simulink model "ISReferenceApplication"  (R2019b)
settings: Solver=VariableStepAuto  StartTime=0.0  StopTime=10.0  RelTol=1e-3
undefined symbols (not defined in the file or in its folder): C_Brake, C_Final, C_Front, C_Middle, C_out_Brake, C_out_Final, C_out_Front, C_out_Middle, Co, Cso, D_out_Brake, D_out_Final, D_out_Front, D_out_Middle, Downshift_Speeds, F, F_Brake, F_Final, F_Front, F_Middle, Fs, G_Brake, G_Final, G_Front, G_Middle, G_sys_Brake, G_sys_Final, G_sys_Front, G_sys_Middle, Gd, Gd_Brake, Gd_Final, Gsd, h, H_Brake, H_Final, H_Front, H_Middle, H_sys_Brake, H_sys_Final, H_sys_Front, H_sys_Middle, Hd, Hd_Brake, Hd_Final, Hsd, JE, JE_Brake, JE_Final, JE_Front, JE_Middle, JEs, JF_part, JF_part_Brake, JF_part_Final, JF_parts, Ld, Ld_Brake, Ld_Final, Ld_Front ... (+21)
libraries: simulink x5, autolibutils x3, sim3dlib x2, vehdynlibviscommon x1
(part 2 of 4)

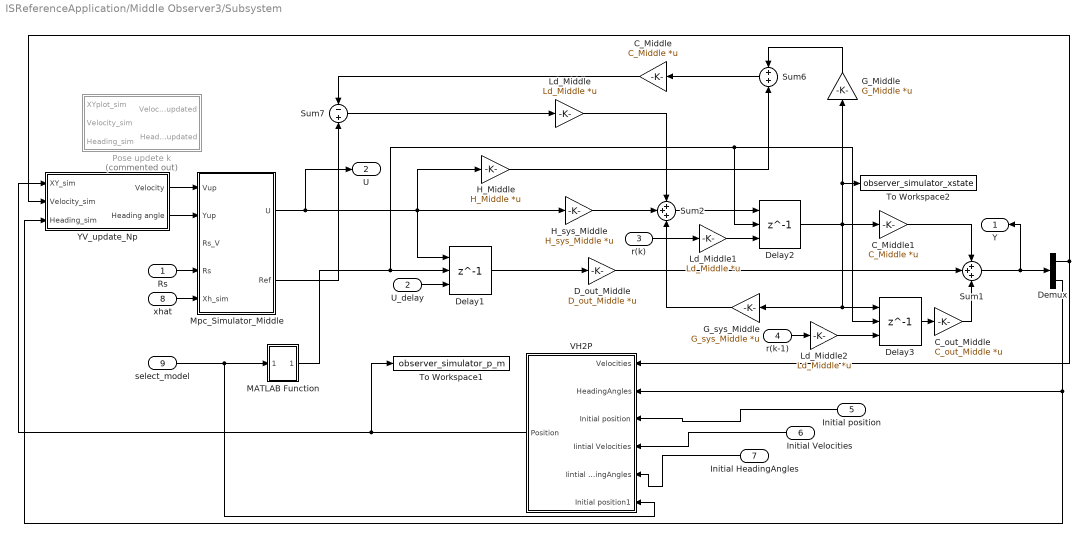
== system ISReferenceApplication/Middle Observer3/Subsystem ==
  Rs : Inport
  U_delay : Inport  Port=2
  r(k) : Inport  Port=3
  r(k-1) : Inport  Port=4
  Initial position : Inport  Port=5
  Initial Velocities : Inport  Port=6
  Initial HeadingAngles : Inport  Port=7
  xhat : Inport  Port=8
  select_model : Inport  Port=9
  C_Middle : Gain  Gain=C_Middle  Multiplication=Matrix(K*u) (u vector)
  C_Middle1 : Gain  Gain=C_Middle  Multiplication=Matrix(K*u) (u vector)
  C_out_Middle : Gain  Gain=C_out_Middle  Multiplication=Matrix(K*u) (u vector)
  D_out_Middle : Gain  Gain=D_out_Middle  Multiplication=Matrix(K*u) (u vector)
  Delay1 : Delay  DelayLength=1  InitialConditionSource=Input port  InitialCondition=0  ExternalReset=Rising  SampleTime=Ts
      settings: InputPortMap=u0,r5,p4
  Delay2 : Delay  DelayLength=1  InitialConditionSource=Input port  InitialCondition=0  ExternalReset=Rising  SampleTime=Ts
      settings: InputPortMap=u0,r5,p4
  Delay3 : Delay  DelayLength=1  InitialConditionSource=Input port  InitialCondition=0  ExternalReset=Rising  SampleTime=Ts
      settings: InputPortMap=u0,r5,p4
  Demux : Demux  Outputs=2
  G_Middle : Gain  Gain=G_Middle  Multiplication=Matrix(K*u) (u vector)
  G_sys_Middle : Gain  Gain=G_sys_Middle  Multiplication=Matrix(K*u) (u vector)
  H_Middle : Gain  Gain=H_Middle  Multiplication=Matrix(K*u) (u vector)
  H_sys_Middle : Gain  Gain=H_sys_Middle  Multiplication=Matrix(K*u) (u vector)
  Ld_Middle : Gain  Gain=Ld_Middle  Multiplication=Matrix(K*u) (u vector)
  Ld_Middle1 : Gain  Gain=Ld_Middle  Multiplication=Matrix(K*u) (u vector)
  Ld_Middle2 : Gain  Gain=Ld_Middle  Multiplication=Matrix(K*u) (u vector)
  MATLAB Function : MATLAB Function  TreatAsAtomicUnit=on
  Mpc_Simulator_Middle : Subsystem
  Pose updete k : Subsystem  Commented=on
  Sum1 : Sum  Inputs=+++
  Sum2 : Sum  Inputs=+++
  Sum6 : Sum
  Sum7 : Sum  Inputs=-+
  To Workspace1 : ToWorkspace  VariableName=observer_simulator_p_m  SampleTime=Ts
  To Workspace2 : ToWorkspace  VariableName=observer_simulator_xstate  SampleTime=Ts
  VH2P : Subsystem
  YV_update_Np : Subsystem  TreatAsAtomicUnit=on
  Y : Outport  VectorParamsAs1DForOutWhenUnconnected=off
  U : Outport  Port=2  VectorParamsAs1DForOutWhenUnconnected=off
  wires:
  MATLAB Function/1(tri) -> Delay1/2, Delay2/2, Delay3/2
  select_model/1 -> MATLAB Function/1(select_model), VH2P/6(Initial position1)
  Initial position/1 -> VH2P/3(Initial position)
  Sum2/1 -> Delay2/1
  Demux/2 -> YV_update_Np/3(Heading_sim), VH2P/2(HeadingAngles)
  Ld_Middle/1 -> Sum2/1
  Sum7/1 -> Ld_Middle/1
  Mpc_Simulator_Middle/2(Ref) -> Sum7/2
  Rs/1 -> Mpc_Simulator_Middle/4(Rs)
  C_out_Middle/1 -> Sum1/3
  G_Middle/1 -> Sum6/1
  C_Middle/1 -> Sum7/1
  Mpc_Simulator_Middle/1(U) -> U/1, H_sys_Middle/1, H_Middle/1, Delay1/1
  H_sys_Middle/1 -> Sum2/2
  G_sys_Middle/1 -> Sum2/3
  Delay3/1 -> C_out_Middle/1
  VH2P/1(Position) -> YV_update_Np/1(XY_sim), To Workspace1/1
  Demux/1 -> YV_update_Np/2(Velocity_sim), VH2P/1(Velocities)
  Delay2/1 -> To Workspace2/1, G_Middle/1, G_sys_Middle/1, Delay3/1, C_Middle1/1
  H_Middle/1 -> Sum6/2
  Sum1/1 -> Y/1, Demux/1
  Sum6/1 -> C_Middle/1
  D_out_Middle/1 -> Sum1/2
  Delay1/1 -> D_out_Middle/1
  C_Middle1/1 -> Sum1/1
  YV_update_Np/2(Heading angle) -> Mpc_Simulator_Middle/2(Yup)
  xhat/1 -> Mpc_Simulator_Middle/5(Xh_sim)
  YV_update_Np/1(Velocity) -> Mpc_Simulator_Middle/1(Vup)
  r(k)/1 -> Ld_Middle1/1
  Ld_Middle1/1 -> Delay2/3
  U_delay/1 -> Delay1/3
  r(k-1)/1 -> Ld_Middle2/1
  Ld_Middle2/1 -> Delay3/3
  Initial Velocities/1 -> VH2P/4(Iintial Velocities)
  Initial HeadingAngles/1 -> VH2P/5(Iintial HeadingAngles)

== system ISReferenceApplication/Passenger Vehicle/Body, Suspension, Wheels ==
  note: 1) Add Subsystem or Model blocks as valid variant choices.
      | 2) You cannot connect blocks at this level. At simulation, connectivity is automatically
      | determined, based on the active variant and port name matching.
  WindXYZ : Inport
  Ground : Inport  Port=2  PortDimensions=4
  Friction : Inport  Port=3  PortDimensions=4
  WhlAng : Inport  Port=4
  AxlTrq : Inport  Port=5
  BrkPrs : Inport  Port=6
  PassVeh14DOF : ModelReference  DisableCoverage=on  ModelNameDialog=PassVeh14DOF  VariantControl=3  ModelReferenceVersion=1.296
  PassVeh7DOF : ModelReference  DisableCoverage=on  ModelNameDialog=PassVeh7DOF  VariantControl=1  ModelReferenceVersion=1.144
  Cgxyzdot : Outport  VectorParamsAs1DForOutWhenUnconnected=off
  CgXYZ : Outport  Port=2  VectorParamsAs1DForOutWhenUnconnected=off
  CgXYZdot : Outport  Port=3  VectorParamsAs1DForOutWhenUnconnected=off
  angles : Outport  Port=4  VectorParamsAs1DForOutWhenUnconnected=off
  pqr : Outport  Port=5  VectorParamsAs1DForOutWhenUnconnected=off
  Cgaxyz : Outport  Port=6  VectorParamsAs1DForOutWhenUnconnected=off
  Beta : Outport  Port=7  VectorParamsAs1DForOutWhenUnconnected=off
  GeomXYZ : Outport  Port=8  VectorParamsAs1DForOutWhenUnconnected=off
  GeomXYZdot : Outport  Port=9  VectorParamsAs1DForOutWhenUnconnected=off
  Omega : Outport  Port=10  PortDimensions=4  VectorParamsAs1DForOutWhenUnconnected=off
  Kappa : Outport  Port=11  PortDimensions=4  VectorParamsAs1DForOutWhenUnconnected=off
  Alpha : Outport  Port=12  PortDimensions=4  VectorParamsAs1DForOutWhenUnconnected=off
  XWheel : Outport  Port=13  VectorParamsAs1DForOutWhenUnconnected=off
  YWheel : Outport  Port=14  VectorParamsAs1DForOutWhenUnconnected=off
  dzWheel : Outport  Port=15  VectorParamsAs1DForOutWhenUnconnected=off

== system ISReferenceApplication/Passenger Vehicle/Engine ==
  note: 1) Add Subsystem or Model blocks as valid variant choices.
      | 2) You cannot connect blocks at this level. At simulation, connectivity is automatically
      | determined, based on the active variant and port name matching.
  TrqCmd : Inport
  EngSpd : Inport  Port=2  Unit=rad/s
  Ideal Mapped Engine : ModelReference  DisableCoverage=on  ModelNameDialog=SiMappedEngineV  VariantControl=0  ModelReferenceVersion=1.324
  EngTrq : Outport  VectorParamsAs1DForOutWhenUnconnected=off

== system ISReferenceApplication/Passenger Vehicle/Steering, Transmission, Driveline and Brakes ==
  note: 1) Add Subsystem or Model blocks as valid variant choices.
      | 2) You cannot connect blocks at this level. At simulation, connectivity is automatically
      | determined, based on the active variant and port name matching.
  SteerHWCmd : Inport
  EngTrq : Inport  Port=2
  GearCmd : Inport  Port=3  OutDataTypeStr=int8
  BrkPrsCmd : Inport  Port=4  PortDimensions=4
  Omega : Inport  Port=5
  DiffPrsCmd : Inport  Port=6
  Driveline Ideal Fixed Gear : ModelReference  DisableCoverage=on  ModelNameDialog=Driveline  VariantControl=0  ModelReferenceVersion=1.216
  WhlAng : Outport  VectorParamsAs1DForOutWhenUnconnected=off
  AxlTrq : Outport  Port=2  VectorParamsAs1DForOutWhenUnconnected=off
  BrkPrs : Outport  Port=3  PortDimensions=4  VectorParamsAs1DForOutWhenUnconnected=off
  EngSpd : Outport  Port=4  Unit=rad/s  VectorParamsAs1DForOutWhenUnconnected=off
  PropShftSpd : Outport  Port=5  VectorParamsAs1DForOutWhenUnconnected=off
  StrWhlTrq : Outport  Port=6  VectorParamsAs1DForOutWhenUnconnected=off

== system ISReferenceApplication/Passenger Vehicle/Subsystem ==
  Env : Inport
  Driveline : Inport  Port=2
  Bus Selector1 : BusSelector  OutputSignals=Gnd.z.G_FL_z,Gnd.z.G_FR_z,Gnd.z.G_RL_z,Gnd.z.G_RR_z
  Bus Selector2 : BusSelector  OutputSignals=Wind
  Bus Selector3 : BusSelector  OutputSignals=Gnd.mu.mu_FL,Gnd.mu.mu_FR,Gnd.mu.mu_RL,Gnd.mu.mu_RR
  Bus Selector4 : BusSelector  OutputSignals=WhlAng,AxlTrq,BrkPrs
  Vector Concatenate : Concatenate  NumInputs=4
  Vector Concatenate1 : Concatenate  NumInputs=4
  Wind : Outport  VectorParamsAs1DForOutWhenUnconnected=off
  Gnd : Outport  Port=2  VectorParamsAs1DForOutWhenUnconnected=off
  mu : Outport  Port=3  VectorParamsAs1DForOutWhenUnconnected=off
  WhlAng : Outport  Port=4  VectorParamsAs1DForOutWhenUnconnected=off
  AxlTrq : Outport  Port=5  VectorParamsAs1DForOutWhenUnconnected=off
  BrkPrs : Outport  Port=6  VectorParamsAs1DForOutWhenUnconnected=off
  wires:
  Bus Selector4/3 -> BrkPrs/1  "<BrkPrs>"
  Bus Selector4/1 -> WhlAng/1  "<WhlAng>"
  Bus Selector4/2 -> AxlTrq/1  "<AxlTrq>"
  Driveline/1 -> Bus Selector4/1
  Vector Concatenate1/1 -> Gnd/1
  Bus Selector1/4 -> Vector Concatenate1/4  "<G_RR_z>"
  Bus Selector1/3 -> Vector Concatenate1/3  "<G_RL_z>"
  Bus Selector1/2 -> Vector Concatenate1/2  "<G_FR_z>"
  Bus Selector1/1 -> Vector Concatenate1/1  "<G_FL_z>"
  Vector Concatenate/1 -> mu/1
  Bus Selector3/4 -> Vector Concatenate/4  "<mu_RR>"
  Bus Selector3/3 -> Vector Concatenate/3  "<mu_RL>"
  Bus Selector3/2 -> Vector Concatenate/2  "<mu_FR>"
  Bus Selector3/1 -> Vector Concatenate/1  "<mu_FL>"
  Bus Selector2/1 -> Wind/1  "<Wind>"
  Env/1 -> Bus Selector2/1, Bus Selector1/1, Bus Selector3/1

== system ISReferenceApplication/Passenger Vehicle/Subsystem1 ==
  WhlAng : Inport
  AxlTrq : Inport  Port=2
  BrkPrs : Inport  Port=3
  EngSpd : Inport  Port=4
  PropShftSpd : Inport  Port=5
  StrWhlTrq : Inport  Port=6
  Bus Creator1 : BusCreator  Inputs=5
  Bus Creator2 : BusCreator  Inputs=1
  Driveline : Outport  VectorParamsAs1DForOutWhenUnconnected=off
  Steering : Outport  Port=2  VectorParamsAs1DForOutWhenUnconnected=off
  wires:
  Bus Creator2/1 -> Steering/1  "Steering"
  StrWhlTrq/1 -> Bus Creator2/1  "StrWhlTrq"
  BrkPrs/1 -> Bus Creator1/3  "BrkPrs"
  EngSpd/1 -> Bus Creator1/4  "EngSpd"
  WhlAng/1 -> Bus Creator1/1  "WhlAng"
  AxlTrq/1 -> Bus Creator1/2  "AxlTrq"
  PropShftSpd/1 -> Bus Creator1/5  "PropShftSpd"
  Bus Creator1/1 -> Driveline/1  "Driveline"

== system ISReferenceApplication/Passenger Vehicle/Subsystem2 ==
  Cntrl : Inport
  SteerCmd : Inport  Port=2
  EngTrqCmd : Inport  Port=3
  Wheels : Inport  Port=4
  Bus Selector1 : BusSelector  OutputSignals=SteerCmd
  Bus Selector2 : BusSelector  OutputSignals=Omega
  Bus Selector3 : BusSelector  OutputSignals=Transmission.GearCmd,Brake.BrkPrsCmd,Diff.DiffPrsCmd
  Bus Selector4 : BusSelector  OutputSignals=EngTrq
  Data Type Conversion : DataTypeConversion
  Steer : Outport  VectorParamsAs1DForOutWhenUnconnected=off
  EngTrq : Outport  Port=2  VectorParamsAs1DForOutWhenUnconnected=off
  GearCmd : Outport  Port=3  VectorParamsAs1DForOutWhenUnconnected=off
  BrkPrsCmd : Outport  Port=4  VectorParamsAs1DForOutWhenUnconnected=off
  Omega : Outport  Port=5  VectorParamsAs1DForOutWhenUnconnected=off
  DiffPrsCmd : Outport  Port=6  VectorParamsAs1DForOutWhenUnconnected=off
  wires:
  Data Type Conversion/1 -> GearCmd/1
  Bus Selector3/3 -> DiffPrsCmd/1  "<DiffPrsCmd>"
  Bus Selector4/1 -> EngTrq/1  "<EngTrq>"
  Bus Selector1/1 -> Steer/1  "<SteerCmd>"
  EngTrqCmd/1 -> Bus Selector4/1
  Bus Selector3/2 -> BrkPrsCmd/1  "<BrkPrsCmd>"
  Bus Selector2/1 -> Omega/1  "<Omega>"
  Wheels/1 -> Bus Selector2/1
  SteerCmd/1 -> Bus Selector1/1
  Bus Selector3/1 -> Data Type Conversion/1  "<GearCmd>"
  Cntrl/1 -> Bus Selector3/1

== system ISReferenceApplication/Passenger Vehicle/Subsystem3 ==
  Cntrl : Inport
  Driveline : Inport  Port=2
  Bus Selector : BusSelector  OutputSignals=ECU.EngTrqCmd
  Bus Selector1 : BusSelector  OutputSignals=EngSpd
  EngTrqCmd : Outport  VectorParamsAs1DForOutWhenUnconnected=off
  EngSpd : Outport  Port=2  VectorParamsAs1DForOutWhenUnconnected=off
  wires:
  Bus Selector1/1 -> EngSpd/1  "<EngSpd>"
  Bus Selector/1 -> EngTrqCmd/1  "<EngTrqCmd>"
  Cntrl/1 -> Bus Selector/1
  Driveline/1 -> Bus Selector1/1

== system ISReferenceApplication/Passenger Vehicle/Subsystem4 ==
  Cgxyzdot : Inport
  CgXYZ : Inport  Port=2
  CgXYZdot : Inport  Port=3
  angles : Inport  Port=4
  pqr : Inport  Port=5
  Cgaxyz : Inport  Port=6
  Beta : Inport  Port=7
  GeomXYZ : Inport  Port=8
  GeomXYZdot : Inport  Port=9
  Omega : Inport  Port=10
  Kappa : Inport  Port=11
  Alpha : Inport  Port=12
  XWheel : Inport  Port=13
  YWheel : Inport  Port=14
  dzWheel : Inport  Port=15
  Bus Creator : BusCreator  Inputs=25
  Bus Creator3 : BusCreator  Inputs=6
  Demux{,1..7} (8 alike) : Demux  Outputs=3
  Chassis : Outport  VectorParamsAs1DForOutWhenUnconnected=off
  Wheels : Outport  Port=2  VectorParamsAs1DForOutWhenUnconnected=off
  wires:
  Demux7/3 -> Bus Creator/25  "GeomZdot"
  Demux7/2 -> Bus Creator/24  "GeomYdot"
  Demux7/1 -> Bus Creator/23  "GeomXdot"
  Demux6/3 -> Bus Creator/22  "GeomZ"
  Demux6/2 -> Bus Creator/21  "GeomY"
  Demux6/1 -> Bus Creator/20  "GeomX"
  Beta/1 -> Bus Creator/19  "Beta"
  Demux5/3 -> Bus Creator/18  "az"
  Demux5/2 -> Bus Creator/17  "ay"
  Demux5/1 -> Bus Creator/16  "ax"
  Demux4/3 -> Bus Creator/15  "r"
  Demux4/2 -> Bus Creator/14  "q"
  Demux4/1 -> Bus Creator/13  "p"
  Demux3/3 -> Bus Creator/12  "psi"
  Demux3/2 -> Bus Creator/11  "theta"
  Demux3/1 -> Bus Creator/10  "phi"
  Demux2/3 -> Bus Creator/9  "Zdot"
  Demux2/2 -> Bus Creator/8  "Ydot"
  Demux2/1 -> Bus Creator/7  "Xdot"
  Demux1/3 -> Bus Creator/6  "Z"
  Demux1/2 -> Bus Creator/5  "Y"
  Demux1/1 -> Bus Creator/4  "X"
  Demux/3 -> Bus Creator/3  "zdot"
  Demux/2 -> Bus Creator/2  "ydot"
  Demux/1 -> Bus Creator/1  "xdot"
  GeomXYZ/1 -> Demux6/1
  GeomXYZdot/1 -> Demux7/1
  Cgaxyz/1 -> Demux5/1
  pqr/1 -> Demux4/1
  angles/1 -> Demux3/1
  CgXYZdot/1 -> Demux2/1
  CgXYZ/1 -> Demux1/1
  Cgxyzdot/1 -> Demux/1
  Alpha/1 -> Bus Creator3/2  "Alpha"
  XWheel/1 -> Bus Creator3/4  "XWheel"
  YWheel/1 -> Bus Creator3/5  "YWheel"
  Bus Creator3/1 -> Wheels/1  "Wheels"
  Kappa/1 -> Bus Creator3/1  "Kappa"
  dzWheel/1 -> Bus Creator3/6  "dZWheel"
  Omega/1 -> Bus Creator3/3  "Omega"
  Bus Creator/1 -> Chassis/1  "Chassis"

== system ISReferenceApplication/Passenger Vehicle/Subsystem5 ==
  "EngTrq " : Inport
  Bus Creator : BusCreator  Inputs=1
  Eng : Outport  VectorParamsAs1DForOutWhenUnconnected=off
  wires:
  Bus Creator/1 -> Eng/1
  "EngTrq "/1 -> Bus Creator/1  "EngTrq"

== system ISReferenceApplication/Visualization/3D Engine ==
  note: 1) Add Subsystem or Model blocks as valid variant choices.
      | 2) You cannot connect blocks at this level. At simulation, connectivity is automatically
      | determined, based on the active variant and port name matching.
  VehFdbk : Inport
  3D Engine : Subsystem  VariantControl=1
  3D Engine Disabled : Subsystem  VariantControl=0

== system ISReferenceApplication/Visualization/Vehicle XY Plotter ==
  VehFdbk : Inport
  Bus Selector1 : BusSelector  OutputSignals=Body.phi,Body.theta,Body.psi  OutputAsBus=on
  Bus Selector2 : BusSelector  OutputSignals=Driveline.WhlAng  OutputAsBus=on
  Bus Selector3 : BusSelector  OutputSignals=Body.X,Body.Y,Body.Z  OutputAsBus=on
  Bus Selector4 : BusSelector  OutputSignals=Body.Xdot,Body.Ydot  OutputAsBus=on
  Bus to Vector{,1..3} (4 alike) : BusToVector
  Ground : Ground
  Rate Transition{1..2,5..6} (4 alike) : RateTransition  OutPortSampleTime=pltDT
  Vector Concatenate : Concatenate
  Vehicle XY Plotter : vehdynlibviscommon/Vehicle XY Plotter  bufferSize=bufferSize  w=w  a=a  b=b  figBorder=figBorder
      settings: SourceProductName=Vehicle Dynamics Blockset  SourceProductBaseCode=VE
  wires:
  Rate Transition2/1 -> Vehicle XY Plotter/4
  VehFdbk/1 -> Bus Selector3/1, Bus Selector4/1, Bus Selector2/1, Bus Selector1/1
  Bus Selector2/1 -> Bus to Vector3/1
  Bus to Vector3/1 -> Rate Transition2/1
  Ground/1 -> Vector Concatenate/2
  Bus to Vector1/1 -> Vector Concatenate/1
  Bus Selector3/1 -> Bus to Vector/1
  Bus to Vector/1 -> Rate Transition5/1  "InertCGDisp"
  Bus Selector1/1 -> Bus to Vector2/1
  Vector Concatenate/1 -> Rate Transition6/1  "InertCGVel"
  Rate Transition6/1 -> Vehicle XY Plotter/3
  Rate Transition1/1 -> Vehicle XY Plotter/2
  Bus Selector4/1 -> Bus to Vector1/1
  Rate Transition5/1 -> Vehicle XY Plotter/1
  Bus to Vector2/1 -> Rate Transition1/1  "InertCGDisp"

== system ISReferenceApplication/Controllers1/Active Differential Control/No Control ==
  YawRate : Inport
  Steer : Inport  Port=2
  Ground : Ground
  Terminator : Terminator
  Terminator1 : Terminator
  Vector Concatenate2 : Concatenate  NumInputs=4
  DiffPrsCmd : Outport  VectorParamsAs1DForOutWhenUnconnected=off
  TrqCmd : Outport  Port=2  VectorParamsAs1DForOutWhenUnconnected=off
  wires:
  YawRate/1 -> Terminator/1
  Vector Concatenate2/1 -> DiffPrsCmd/1  "Reference P"
  Steer/1 -> Terminator1/1
  Ground/1 -> Vector Concatenate2/2, Vector Concatenate2/3, Vector Concatenate2/4, TrqCmd/1, Vector Concatenate2/1

== system ISReferenceApplication/Controllers1/Active Differential Control/Rear Diff Controller ==
  YawRate : Inport
  Steer : Inport  Port=2
  Abs : Abs  ZeroCross=off
  Abs1 : Abs  ZeroCross=off
  Cont LPF : autolibutils/Cont LPF  wc=10*pi  aMode=2
      settings: SourceProductName=Powertrain Blockset  SourceProductBaseCode=PW
  Cont LPF1 : autolibutils/Cont LPF  wc=1*pi  aMode=2
      settings: SourceProductName=Powertrain Blockset  SourceProductBaseCode=PW
  Dead Zone : DeadZone  LowerValue=-.01  UpperValue=.01  ZeroCross=off  SaturateOnIntegerOverflow=on
  Gain : Gain  Gain=1e6
  Gain2 : Gain  Gain=1/4
  Gain3 : Gain  Gain=2e3
  Ground : Ground
  Saturation : Saturate  UpperLimit=0  LowerLimit=-inf  ZeroCross=off
  Saturation1 : Saturate  UpperLimit=inf  LowerLimit=0  ZeroCross=off
  Saturation2 : Saturate  UpperLimit=1e7  LowerLimit=0  ZeroCross=off
  Saturation3 : Saturate  UpperLimit=200  LowerLimit=0  ZeroCross=off
  Subtract : Sum  Inputs=+-
  Vector Concatenate2 : Concatenate  NumInputs=4
  DiffPrsCmd : Outport  VectorParamsAs1DForOutWhenUnconnected=off
  TrqCmd : Outport  Port=2  VectorParamsAs1DForOutWhenUnconnected=off
  wires:
  Cont LPF1/1 -> Abs1/1
  Dead Zone/1 -> Cont LPF/1, Cont LPF1/1
  Saturation3/1 -> TrqCmd/1
  Saturation2/1 -> DiffPrsCmd/1
  Cont LPF/1 -> Saturation/1, Saturation1/1
  Abs1/1 -> Gain3/1
  Subtract/1 -> Dead Zone/1
  YawRate/1 -> Subtract/1
  Gain2/1 -> Subtract/2
  Gain3/1 -> Saturation3/1
  Abs/1 -> Vector Concatenate2/3
  Gain/1 -> Saturation2/1
  Saturation1/1 -> Vector Concatenate2/4
  Saturation/1 -> Abs/1
  Steer/1 -> Gain2/1
  Ground/1 -> Vector Concatenate2/1, Vector Concatenate2/2
  Vector Concatenate2/1 -> Gain/1  "Reference P"

== system ISReferenceApplication/Controllers1/Brake Controller/Brake Pressure Control ==
  note: 1) Add Subsystem or Model blocks as valid variant choices.
      | 2) You cannot connect blocks at this level. At simulation, connectivity is automatically
      | determined, based on the active variant and port name matching.
  Pref : Inport
  xdot : Inport  Port=2
  <Kappa> : Inport  Port=3
  Bang Bang ABS : Subsystem  VariantControl=1
  Open Loop : Subsystem  VariantControl=0
  PCmd : Outport  VectorParamsAs1DForOutWhenUnconnected=off

== system ISReferenceApplication/Controllers1/Transmission Controller/TCM ==
  AccCmd : Inport
  EngSpd : Inport  Port=2
  VehSpdFdbk : Inport  Port=3
  function : TriggerPort  TriggerType=function-call  VariantControl=Variant
  Neutral Select : Subsystem
  Prop Shaft Speed LPF : DiscreteTransferFcn  Numerator=[0.000000000000000 0.009950166250832 ]  Denominator=[1.000000000000000 -0.990049833749168 ]  mask(DiscretizedDiscreteTransferFcn){}
      mask init:
      | %zoh
  TCM Shift Controller : Stateflow chart  TreatAsAtomicUnit=on
  prop speed to vehicle speed : Gain  Gain=0.45
  Gear Select : Outport  VectorParamsAs1DForOutWhenUnconnected=off
  wires:
  Prop Shaft Speed LPF/1 -> prop speed to vehicle speed/1
  prop speed to vehicle speed/1 -> TCM Shift Controller/1(speed)
  EngSpd/1 -> Neutral Select/2(EngSpd)
  Neutral Select/1(Neutral Select) -> TCM Shift Controller/3(Neutral)
  AccCmd/1 -> TCM Shift Controller/2(pedal), Neutral Select/1(AccCmd)  "AccCmd"
  TCM Shift Controller/1(GearState) -> Gear Select/1  "GearCmd"
  VehSpdFdbk/1 -> Prop Shaft Speed LPF/1

== system ISReferenceApplication/Final Observer1/Subsystem/Mpc_Simulator_Final ==
  Vup : Inport  SampleTime=Ts  LockScale=on
  Yup : Inport  Port=2  SampleTime=Ts  LockScale=on
  Rs : Inport  Port=3  SampleTime=Ts  LockScale=on
  Xh_sim : Inport  Port=4
  Clock : Clock
  Constant1 : Constant  Value=M  VectorParams1D=off  SampleTime=-1
  Constant2 : Constant  Value=Np  SampleTime=-1
  Constant4 : Constant  Value=Qc  VectorParams1D=off  SampleTime=-1
  Constant5 : Constant  Value=phi_Brake  VectorParams1D=off  SampleTime=-1
  Constant6 : Constant  Value=JE_Brake  VectorParams1D=off  SampleTime=-1
  Constant7 : Constant  Value=Upd_end  VectorParams1D=off  SampleTime=-1
  F_Final : Gain  Gain=F_Brake  Multiplication=Matrix(K*u) (u vector)
  MATLAB Function : MATLAB Function  TreatAsAtomicUnit=on  SystemSampleTime=Ts
  Unit Delay : UnitDelay  InitialCondition=[0;0]  SampleTime=Ts  HasFrameUpgradeWarning=on
  U : Outport  VectorParamsAs1DForOutWhenUnconnected=off
  Ref : Outport  Port=2  VectorParamsAs1DForOutWhenUnconnected=off
  wires:
  Unit Delay/1 -> MATLAB Function/12(u)
  MATLAB Function/2(U) -> Unit Delay/1, U/1
  MATLAB Function/1(Ref) -> Ref/1
  Xh_sim/1 -> F_Final/1
  Constant4/1 -> MATLAB Function/5(Qc)
  Constant5/1 -> MATLAB Function/4(phi)
  Constant6/1 -> MATLAB Function/1(JE)
  Constant2/1 -> MATLAB Function/3(Np)
  Yup/1 -> MATLAB Function/7(Yup)
  Constant1/1 -> MATLAB Function/2(M)
  Clock/1 -> MATLAB Function/10(Tsim)
  F_Final/1 -> MATLAB Function/6(Fxh)
  Vup/1 -> MATLAB Function/8(Vup)
  Rs/1 -> MATLAB Function/9(Rs)
  Constant7/1 -> MATLAB Function/11(Upd_end)

== system ISReferenceApplication/Final Observer1/Subsystem/Pose updete k ==
  XYplot_sim : Inport
  Velocity_sim : Inport  Port=2
  Heading_sim : Inport  Port=3
  Clock : Clock
  From Workspace : FromWorkspace  VariableName=Rs_V_now  SampleTime=Ts
  From Workspace1 : FromWorkspace  VariableName=Rs_Y_now  SampleTime=Ts
  From Workspace2 : FromWorkspace  VariableName=XYplot_X  SampleTime=Ts
  From Workspace3 : FromWorkspace  VariableName=XYplot_Y  SampleTime=Ts
  Mux : Mux  Inputs=2
  Reshape : Reshape  OutputDimensionality=Customize  OutputDimensions=[pick_num,2]
  Trajectroy : Constant  Value=XYplot  VectorParams1D=off  SampleTime=-1
  Unit Delay{,1..3} (4 alike) : UnitDelay  SampleTime=Ts  HasFrameUpgradeWarning=on
  Update : MATLAB Function  TreatAsAtomicUnit=on  SystemSampleTime=Ts
      settings: RTWFcnNameOpts=Use subsystem name
  Velocity_updated : Outport  VectorParamsAs1DForOutWhenUnconnected=off
  Heading_updated : Outport  Port=2  VectorParamsAs1DForOutWhenUnconnected=off
  wires:
  XYplot_sim/1 -> Update/5(XYplot_sim), Unit Delay3/1
  Heading_sim/1 -> Unit Delay2/1, Update/9(Heading_sim)
  Clock/1 -> Update/11(Tsim)
  Velocity_sim/1 -> Update/7(Velocity_sim), Unit Delay1/1
  Update/2(Heading_updated) -> Heading_updated/1
  Update/1(Velocity_updated) -> Velocity_updated/1
  From Workspace/1 -> Update/1(Rs_V_now)
  Update/3(Heading_end) -> Unit Delay/1
  Unit Delay/1 -> Update/12(Last_Heading_end)
  From Workspace1/1 -> Update/2(Rs_Y_now)
  Unit Delay1/1 -> Update/8(Last_Velocity_sim)
  Unit Delay2/1 -> Update/10(Last_Heading_sim)
  Unit Delay3/1 -> Update/6(Last_XYplot_sim)
  Mux/1 -> Reshape/1
  From Workspace2/1 -> Mux/1
  From Workspace3/1 -> Mux/2
  Trajectroy/1 -> Update/3(XYline)
  Reshape/1 -> Update/4(XYplot)

== system ISReferenceApplication/Final Observer1/Subsystem/VH2P ==
  Velocities : Inport
  HeadingAngles : Inport  Port=2
  Initial position : Inport  Port=3
  Iintial Velocities : Inport  Port=4
  Iintial HeadingAngles : Inport  Port=5
  select_model : Inport  Port=6
  From Workspace : FromWorkspace  VariableName=T_sim  SampleTime=Ts
  MATLAB Function1 : MATLAB Function  TreatAsAtomicUnit=on
  Resettable Delay : Delay  DelayLength=1  InitialConditionSource=Input port  ExternalReset=Rising  SampleTime=Ts
      settings: InputPortMap=u0,r5,p4
  Resettable Delay1 : Delay  DelayLength=1  InitialConditionSource=Input port  ExternalReset=Rising  SampleTime=Ts
      settings: InputPortMap=u0,r5,p4
  Resettable Delay2 : Delay  DelayLength=1  InitialConditionSource=Input port  ExternalReset=Rising  SampleTime=Ts
      settings: InputPortMap=u0,r5,p4
  Unit Delay3 : UnitDelay  SampleTime=Ts  HasFrameUpgradeWarning=on
  YV2P : MATLAB Function  TreatAsAtomicUnit=on  SystemSampleTime=Ts
  Position : Outport  VectorParamsAs1DForOutWhenUnconnected=off
  wires:
  YV2P/1(Position) -> Resettable Delay/1, Position/1
  Velocities/1 -> Resettable Delay1/1, YV2P/1(Velocity)
  Resettable Delay1/1 -> YV2P/3(LastVelocity)
  HeadingAngles/1 -> YV2P/2(Yaw), Resettable Delay2/1
  Resettable Delay2/1 -> YV2P/4(LastYaw)
  Resettable Delay/1 -> YV2P/7(Lastpostion)
  Initial position/1 -> Resettable Delay/3
  Iintial Velocities/1 -> Resettable Delay1/3
  Iintial HeadingAngles/1 -> Resettable Delay2/3
  Unit Delay3/1 -> YV2P/6(LastTsim)
  From Workspace/1 -> Unit Delay3/1, YV2P/5(Tsim)
  select_model/1 -> MATLAB Function1/1(select_model)
  MATLAB Function1/1(tri) -> Resettable Delay1/2, Resettable Delay2/2, Resettable Delay/2

== system ISReferenceApplication/Final Observer1/Subsystem/YV_update_Np ==
  XY_sim : Inport
  Velocity_sim : Inport  Port=2
  Heading_sim : Inport  Port=3
  From Workspace1 : FromWorkspace  VariableName=T_sim  SampleTime=Ts
  From Workspace3 : FromWorkspace  VariableName=XY_Ref_Upd  SampleTime=Ts
  MATLAB Function2 : MATLAB Function  TreatAsAtomicUnit=on  SystemSampleTime=Ts
  Unit Delay1 : UnitDelay  SampleTime=Ts  HasFrameUpgradeWarning=on
  Unit Delay4 : UnitDelay  SampleTime=Ts  HasFrameUpgradeWarning=on
  Unit Delay5 : UnitDelay  SampleTime=Ts  HasFrameUpgradeWarning=on
  Velocity : Outport  VectorParamsAs1DForOutWhenUnconnected=off
  Heading angle : Outport  Port=2  VectorParamsAs1DForOutWhenUnconnected=off
  wires:
  MATLAB Function2/1(Velocity_updated) -> Velocity/1
  From Workspace3/1 -> MATLAB Function2/1(XY_ref)
  MATLAB Function2/2(Heading_updated) -> Heading angle/1
  From Workspace1/1 -> MATLAB Function2/8(Tsim)
  XY_sim/1 -> Unit Delay1/1, MATLAB Function2/2(XY_sim)
  Velocity_sim/1 -> MATLAB Function2/4(Velocity_sim), Unit Delay5/1
  Heading_sim/1 -> MATLAB Function2/6(Yaw_sim), Unit Delay4/1
  Unit Delay1/1 -> MATLAB Function2/3(LastXY_sim)
  Unit Delay5/1 -> MATLAB Function2/5(LastVelocity_sim)
  Unit Delay4/1 -> MATLAB Function2/7(LastYaw_sim)

== system ISReferenceApplication/Final Observer2/Subsystem/Mpc_Simulator_Final ==
  Vup : Inport  SampleTime=Ts  LockScale=on
  Yup : Inport  Port=2  SampleTime=Ts  LockScale=on
  Rs : Inport  Port=3  SampleTime=Ts  LockScale=on
  Xh_sim : Inport  Port=4
  Clock : Clock
  Constant1 : Constant  Value=M  VectorParams1D=off  SampleTime=-1
  Constant2 : Constant  Value=Np  SampleTime=-1
  Constant3 : Constant  Value=Upd_flag  VectorParams1D=off  SampleTime=-1
  Constant4 : Constant  Value=Qc  VectorParams1D=off  SampleTime=-1
  Constant5 : Constant  Value=phi_Final  VectorParams1D=off  SampleTime=-1
  Constant6 : Constant  Value=JE_Final  VectorParams1D=off  SampleTime=-1
  Constant7 : Constant  Value=Upd_end  VectorParams1D=off  SampleTime=-1
  Constant8 : Constant  Value=Timetochange  VectorParams1D=off  SampleTime=-1
  F_Final : Gain  Gain=F_Final  Multiplication=Matrix(K*u) (u vector)
  MATLAB Function : MATLAB Function  TreatAsAtomicUnit=on  SystemSampleTime=Ts
  Unit Delay : UnitDelay  InitialCondition=[0;0]  SampleTime=Ts  HasFrameUpgradeWarning=on
  U : Outport  VectorParamsAs1DForOutWhenUnconnected=off
  Ref : Outport  Port=2  VectorParamsAs1DForOutWhenUnconnected=off
  wires:
  Constant8/1 -> MATLAB Function/2(Timetochange)
  Constant7/1 -> MATLAB Function/13(Upd_end)
  Constant3/1 -> MATLAB Function/1(Upd_flag)
  Rs/1 -> MATLAB Function/11(Rs)
  Vup/1 -> MATLAB Function/10(Vup)
  F_Final/1 -> MATLAB Function/8(Fxh)
  Clock/1 -> MATLAB Function/12(Tsim)
  Constant1/1 -> MATLAB Function/4(M)
  Yup/1 -> MATLAB Function/9(Yup)
  Constant2/1 -> MATLAB Function/5(Np)
  Constant6/1 -> MATLAB Function/3(JE)
  Constant5/1 -> MATLAB Function/6(phi)
  Constant4/1 -> MATLAB Function/7(Qc)
  Xh_sim/1 -> F_Final/1
  MATLAB Function/1(Ref) -> Ref/1
  MATLAB Function/2(U) -> U/1, Unit Delay/1
  Unit Delay/1 -> MATLAB Function/14(u)

== system ISReferenceApplication/Final Observer2/Subsystem/Pose updete k ==
  XYplot_sim : Inport
  Velocity_sim : Inport  Port=2
  Heading_sim : Inport  Port=3
  Clock : Clock
  From Workspace : FromWorkspace  VariableName=Rs_V_now  SampleTime=Ts
  From Workspace1 : FromWorkspace  VariableName=Rs_Y_now  SampleTime=Ts
  From Workspace2 : FromWorkspace  VariableName=XYplot_X  SampleTime=Ts
  From Workspace3 : FromWorkspace  VariableName=XYplot_Y  SampleTime=Ts
  Mux : Mux  Inputs=2
  Reshape : Reshape  OutputDimensionality=Customize  OutputDimensions=[pick_num,2]
  Trajectroy : Constant  Value=XYplot  VectorParams1D=off  SampleTime=-1
  Unit Delay{,1..3} (4 alike) : UnitDelay  SampleTime=Ts  HasFrameUpgradeWarning=on
  Update : MATLAB Function  TreatAsAtomicUnit=on  SystemSampleTime=Ts
      settings: RTWFcnNameOpts=Use subsystem name
  Velocity_updated : Outport  VectorParamsAs1DForOutWhenUnconnected=off
  Heading_updated : Outport  Port=2  VectorParamsAs1DForOutWhenUnconnected=off
  wires:
  Reshape/1 -> Update/4(XYplot)
  Trajectroy/1 -> Update/3(XYline)
  From Workspace3/1 -> Mux/2
  From Workspace2/1 -> Mux/1
  Mux/1 -> Reshape/1
  Unit Delay3/1 -> Update/6(Last_XYplot_sim)
  Unit Delay2/1 -> Update/10(Last_Heading_sim)
  Unit Delay1/1 -> Update/8(Last_Velocity_sim)
  From Workspace1/1 -> Update/2(Rs_Y_now)
  Unit Delay/1 -> Update/12(Last_Heading_end)
  Update/3(Heading_end) -> Unit Delay/1
  From Workspace/1 -> Update/1(Rs_V_now)
  Update/1(Velocity_updated) -> Velocity_updated/1
  Update/2(Heading_updated) -> Heading_updated/1
  Velocity_sim/1 -> Unit Delay1/1, Update/7(Velocity_sim)
  Clock/1 -> Update/11(Tsim)
  Heading_sim/1 -> Update/9(Heading_sim), Unit Delay2/1
  XYplot_sim/1 -> Unit Delay3/1, Update/5(XYplot_sim)

== system ISReferenceApplication/Final Observer2/Subsystem/VH2P ==
  Velocities : Inport
  HeadingAngles : Inport  Port=2
  Initial position : Inport  Port=3
  Iintial Velocities : Inport  Port=4
  Iintial HeadingAngles : Inport  Port=5
  select_model : Inport  Port=6
  From Workspace : FromWorkspace  VariableName=T_sim  SampleTime=Ts
  MATLAB Function1 : MATLAB Function  TreatAsAtomicUnit=on
  Resettable Delay : Delay  DelayLength=1  InitialConditionSource=Input port  ExternalReset=Rising  SampleTime=Ts
      settings: InputPortMap=u0,r5,p4
  Resettable Delay1 : Delay  DelayLength=1  InitialConditionSource=Input port  ExternalReset=Rising  SampleTime=Ts
      settings: InputPortMap=u0,r5,p4
  Resettable Delay2 : Delay  DelayLength=1  InitialConditionSource=Input port  ExternalReset=Rising  SampleTime=Ts
      settings: InputPortMap=u0,r5,p4
  Unit Delay3 : UnitDelay  SampleTime=Ts  HasFrameUpgradeWarning=on
  YV2P : MATLAB Function  TreatAsAtomicUnit=on  SystemSampleTime=Ts
  Position : Outport  VectorParamsAs1DForOutWhenUnconnected=off
  wires:
  MATLAB Function1/1(tri) -> Resettable Delay/2, Resettable Delay2/2, Resettable Delay1/2
  select_model/1 -> MATLAB Function1/1(select_model)
  From Workspace/1 -> YV2P/5(Tsim), Unit Delay3/1
  Unit Delay3/1 -> YV2P/6(LastTsim)
  Iintial HeadingAngles/1 -> Resettable Delay2/3
  Iintial Velocities/1 -> Resettable Delay1/3
  Initial position/1 -> Resettable Delay/3
  Resettable Delay/1 -> YV2P/7(Lastpostion)
  Resettable Delay2/1 -> YV2P/4(LastYaw)
  HeadingAngles/1 -> Resettable Delay2/1, YV2P/2(Yaw)
  Resettable Delay1/1 -> YV2P/3(LastVelocity)
  Velocities/1 -> YV2P/1(Velocity), Resettable Delay1/1
  YV2P/1(Position) -> Position/1, Resettable Delay/1

== system ISReferenceApplication/Final Observer2/Subsystem/YV_update_Np ==
  XY_sim : Inport
  Velocity_sim : Inport  Port=2
  Heading_sim : Inport  Port=3
  From Workspace1 : FromWorkspace  VariableName=T_sim  SampleTime=Ts
  From Workspace3 : FromWorkspace  VariableName=XY_Ref_Upd  SampleTime=Ts
  MATLAB Function2 : MATLAB Function  TreatAsAtomicUnit=on  SystemSampleTime=Ts
  Unit Delay1 : UnitDelay  SampleTime=Ts  HasFrameUpgradeWarning=on
  Unit Delay4 : UnitDelay  SampleTime=Ts  HasFrameUpgradeWarning=on
  Unit Delay5 : UnitDelay  SampleTime=Ts  HasFrameUpgradeWarning=on
  Velocity : Outport  VectorParamsAs1DForOutWhenUnconnected=off
  Heading angle : Outport  Port=2  VectorParamsAs1DForOutWhenUnconnected=off
  wires:
  Unit Delay4/1 -> MATLAB Function2/7(LastYaw_sim)
  Unit Delay5/1 -> MATLAB Function2/5(LastVelocity_sim)
  Unit Delay1/1 -> MATLAB Function2/3(LastXY_sim)
  Heading_sim/1 -> Unit Delay4/1, MATLAB Function2/6(Yaw_sim)
  Velocity_sim/1 -> Unit Delay5/1, MATLAB Function2/4(Velocity_sim)
  XY_sim/1 -> MATLAB Function2/2(XY_sim), Unit Delay1/1
  From Workspace1/1 -> MATLAB Function2/8(Tsim)
  MATLAB Function2/2(Heading_updated) -> Heading angle/1
  From Workspace3/1 -> MATLAB Function2/1(XY_ref)
  MATLAB Function2/1(Velocity_updated) -> Velocity/1

== system ISReferenceApplication/Middle Observer2/Subsystem/Mpc_Simulator_Middle ==
  Vup : Inport  SampleTime=Ts  LockScale=on
  Yup : Inport  Port=2  SampleTime=Ts  LockScale=on
  Rs : Inport  Port=3  SampleTime=Ts  LockScale=on
  Xh_sim : Inport  Port=4
  Clock : Clock
  Constant1 : Constant  Value=M  VectorParams1D=off  SampleTime=-1
  Constant2 : Constant  Value=Np  SampleTime=-1
  Constant3 : Constant  Value=Upd_flag  VectorParams1D=off  SampleTime=-1
  Constant4 : Constant  Value=Qc  VectorParams1D=off  SampleTime=-1
  Constant5 : Constant  Value=phi_Front  VectorParams1D=off  SampleTime=-1
  Constant6 : Constant  Value=JE_Front  VectorParams1D=off  SampleTime=-1
  Constant7 : Constant  Value=Upd_end  VectorParams1D=off  SampleTime=-1
  Constant8 : Constant  Value=Timetochange  VectorParams1D=off  SampleTime=-1
  F_Middle : Gain  Gain=F_Front  Multiplication=Matrix(K*u) (u vector)
  MATLAB Function : MATLAB Function  TreatAsAtomicUnit=on  SystemSampleTime=Ts
  Unit Delay : UnitDelay  InitialCondition=[0;0]  SampleTime=Ts  HasFrameUpgradeWarning=on
  U : Outport  VectorParamsAs1DForOutWhenUnconnected=off
  Ref : Outport  Port=2  VectorParamsAs1DForOutWhenUnconnected=off
  wires:
  Constant8/1 -> MATLAB Function/2(Timetochange)
  Constant7/1 -> MATLAB Function/13(Upd_end)
  Constant3/1 -> MATLAB Function/1(Upd_flag)
  Rs/1 -> MATLAB Function/11(Rs)
  Vup/1 -> MATLAB Function/10(Vup)
  F_Middle/1 -> MATLAB Function/8(Fxh)
  Clock/1 -> MATLAB Function/12(Tsim)
  Constant1/1 -> MATLAB Function/4(M)
  Yup/1 -> MATLAB Function/9(Yup)
  Constant2/1 -> MATLAB Function/5(Np)
  Constant6/1 -> MATLAB Function/3(JE)
  Constant5/1 -> MATLAB Function/6(phi)
  Constant4/1 -> MATLAB Function/7(Qc)
  Xh_sim/1 -> F_Middle/1
  MATLAB Function/1(Ref) -> Ref/1
  MATLAB Function/2(U) -> U/1, Unit Delay/1
  Unit Delay/1 -> MATLAB Function/14(u)

== system ISReferenceApplication/Middle Observer2/Subsystem/Pose updete k ==
  XYplot_sim : Inport
  Velocity_sim : Inport  Port=2
  Heading_sim : Inport  Port=3
  Clock : Clock
  From Workspace : FromWorkspace  VariableName=Rs_V_now  SampleTime=Ts
  From Workspace1 : FromWorkspace  VariableName=Rs_Y_now  SampleTime=Ts
  From Workspace2 : FromWorkspace  VariableName=XYplot_X  SampleTime=Ts
  From Workspace3 : FromWorkspace  VariableName=XYplot_Y  SampleTime=Ts
  Mux : Mux  Inputs=2
  Reshape : Reshape  OutputDimensionality=Customize  OutputDimensions=[pick_num,2]
  Trajectroy : Constant  Value=XYplot  VectorParams1D=off  SampleTime=-1
  Unit Delay{,1..3} (4 alike) : UnitDelay  SampleTime=Ts  HasFrameUpgradeWarning=on
  Update : MATLAB Function  TreatAsAtomicUnit=on  SystemSampleTime=Ts
      settings: RTWFcnNameOpts=Use subsystem name
  Velocity_updated : Outport  VectorParamsAs1DForOutWhenUnconnected=off
  Heading_updated : Outport  Port=2  VectorParamsAs1DForOutWhenUnconnected=off
  wires:
  Reshape/1 -> Update/4(XYplot)
  Trajectroy/1 -> Update/3(XYline)
  From Workspace3/1 -> Mux/2
  From Workspace2/1 -> Mux/1
  Mux/1 -> Reshape/1
  Unit Delay3/1 -> Update/6(Last_XYplot_sim)
  Unit Delay2/1 -> Update/10(Last_Heading_sim)
  Unit Delay1/1 -> Update/8(Last_Velocity_sim)
  From Workspace1/1 -> Update/2(Rs_Y_now)
  Unit Delay/1 -> Update/12(Last_Heading_end)
  Update/3(Heading_end) -> Unit Delay/1
  From Workspace/1 -> Update/1(Rs_V_now)
  Update/1(Velocity_updated) -> Velocity_updated/1
  Update/2(Heading_updated) -> Heading_updated/1
  Velocity_sim/1 -> Unit Delay1/1, Update/7(Velocity_sim)
  Clock/1 -> Update/11(Tsim)
  Heading_sim/1 -> Update/9(Heading_sim), Unit Delay2/1
  XYplot_sim/1 -> Unit Delay3/1, Update/5(XYplot_sim)

== system ISReferenceApplication/Middle Observer2/Subsystem/VH2P ==
  Velocities : Inport
  HeadingAngles : Inport  Port=2
  Initial position : Inport  Port=3
  Iintial Velocities : Inport  Port=4
  Iintial HeadingAngles : Inport  Port=5
  select_model : Inport  Port=6
  Delay1 : Delay  DelayLength=1  InitialConditionSource=Input port  InitialCondition=0  ExternalReset=Rising  SampleTime=Ts
      settings: InputPortMap=u0,r5,p4
  Delay2 : Delay  DelayLength=1  InitialConditionSource=Input port  InitialCondition=0  ExternalReset=Rising  SampleTime=Ts
      settings: InputPortMap=u0,r5,p4
  Delay3 : Delay  DelayLength=1  InitialConditionSource=Input port  InitialCondition=0  ExternalReset=Rising  SampleTime=Ts
      settings: InputPortMap=u0,r5,p4
  From Workspace : FromWorkspace  VariableName=T_sim  SampleTime=Ts
  MATLAB Function1 : MATLAB Function  TreatAsAtomicUnit=on
  Unit Delay3 : UnitDelay  SampleTime=Ts  HasFrameUpgradeWarning=on
  YV2P : MATLAB Function  TreatAsAtomicUnit=on  SystemSampleTime=Ts
  Position : Outport  VectorParamsAs1DForOutWhenUnconnected=off
  wires:
  MATLAB Function1/1(tri) -> Delay2/2, Delay3/2, Delay1/2
  select_model/1 -> MATLAB Function1/1(select_model)
  From Workspace/1 -> YV2P/5(Tsim), Unit Delay3/1
  Iintial HeadingAngles/1 -> Delay3/3
  Iintial Velocities/1 -> Delay1/3
  Initial position/1 -> Delay2/3
  Delay2/1 -> YV2P/7(Lastpostion)
  Delay3/1 -> YV2P/4(LastYaw)
  HeadingAngles/1 -> YV2P/2(Yaw), Delay3/1
  Delay1/1 -> YV2P/3(LastVelocity)
  Velocities/1 -> YV2P/1(Velocity), Delay1/1
  Unit Delay3/1 -> YV2P/6(LastTsim)
  YV2P/1(Position) -> Position/1, Delay2/1

== system ISReferenceApplication/Middle Observer2/Subsystem/YV_update_Np ==
  XY_sim : Inport
  Velocity_sim : Inport  Port=2
  Heading_sim : Inport  Port=3
  From Workspace1 : FromWorkspace  VariableName=T_sim  SampleTime=Ts
  From Workspace3 : FromWorkspace  VariableName=XY_Ref_Upd  SampleTime=Ts
  MATLAB Function2 : MATLAB Function  TreatAsAtomicUnit=on  SystemSampleTime=Ts
  Unit Delay1 : UnitDelay  SampleTime=Ts  HasFrameUpgradeWarning=on
  Unit Delay4 : UnitDelay  SampleTime=Ts  HasFrameUpgradeWarning=on
  Unit Delay5 : UnitDelay  SampleTime=Ts  HasFrameUpgradeWarning=on
  Velocity : Outport  VectorParamsAs1DForOutWhenUnconnected=off
  Heading angle : Outport  Port=2  VectorParamsAs1DForOutWhenUnconnected=off
  wires:
  Unit Delay4/1 -> MATLAB Function2/7(LastYaw_sim)
  Unit Delay5/1 -> MATLAB Function2/5(LastVelocity_sim)
  Unit Delay1/1 -> MATLAB Function2/3(LastXY_sim)
  Heading_sim/1 -> Unit Delay4/1, MATLAB Function2/6(Yaw_sim)
  Velocity_sim/1 -> Unit Delay5/1, MATLAB Function2/4(Velocity_sim)
  XY_sim/1 -> MATLAB Function2/2(XY_sim), Unit Delay1/1
  From Workspace1/1 -> MATLAB Function2/8(Tsim)
  MATLAB Function2/2(Heading_updated) -> Heading angle/1
  From Workspace3/1 -> MATLAB Function2/1(XY_ref)
  MATLAB Function2/1(Velocity_updated) -> Velocity/1

== system ISReferenceApplication/Middle Observer3/Subsystem/Mpc_Simulator_Middle ==
  Vup : Inport  SampleTime=Ts  LockScale=on
  Yup : Inport  Port=2  SampleTime=Ts  LockScale=on
  Rs_V : Inport  Port=3  SampleTime=Ts  LockScale=on
  Rs : Inport  Port=4  SampleTime=Ts  LockScale=on
  Xh_sim : Inport  Port=5
  Clock : Clock
  Constant1 : Constant  Value=M  VectorParams1D=off  SampleTime=-1
  Constant2 : Constant  Value=Np  SampleTime=-1
  Constant3 : Constant  Value=Upd_flag  VectorParams1D=off  SampleTime=-1
  Constant4 : Constant  Value=Qc  VectorParams1D=off  SampleTime=-1
  Constant5 : Constant  Value=phi_Middle  VectorParams1D=off  SampleTime=-1
  Constant6 : Constant  Value=JE_Middle  VectorParams1D=off  SampleTime=-1
  Constant7 : Constant  Value=Upd_end  VectorParams1D=off  SampleTime=-1
  Constant8 : Constant  Value=Timetochange  VectorParams1D=off  SampleTime=-1
  F_Middle : Gain  Gain=F_Middle  Multiplication=Matrix(K*u) (u vector)
  MATLAB Function : MATLAB Function  TreatAsAtomicUnit=on  SystemSampleTime=Ts
  Unit Delay : UnitDelay  InitialCondition=[0;0]  SampleTime=Ts  HasFrameUpgradeWarning=on
  U : Outport  VectorParamsAs1DForOutWhenUnconnected=off
  Ref : Outport  Port=2  VectorParamsAs1DForOutWhenUnconnected=off
  wires:
  Unit Delay/1 -> MATLAB Function/15(u)
  MATLAB Function/2(U) -> Unit Delay/1, U/1
  MATLAB Function/1(Ref) -> Ref/1
  Xh_sim/1 -> F_Middle/1
  Constant4/1 -> MATLAB Function/7(Qc)
  Constant5/1 -> MATLAB Function/6(phi)
  Constant6/1 -> MATLAB Function/3(JE)
  Constant2/1 -> MATLAB Function/5(Np)
  Rs_V/1 -> MATLAB Function/12(Rs_V)
  Yup/1 -> MATLAB Function/9(Yup)
  Constant1/1 -> MATLAB Function/4(M)
  Clock/1 -> MATLAB Function/13(Tsim)
  F_Middle/1 -> MATLAB Function/8(Fxh)
  Vup/1 -> MATLAB Function/10(Vup)
  Rs/1 -> MATLAB Function/11(Rs)
  Constant3/1 -> MATLAB Function/1(Upd_flag)
  Constant7/1 -> MATLAB Function/14(Upd_end)
  Constant8/1 -> MATLAB Function/2(Timetochange)

== system ISReferenceApplication/Middle Observer3/Subsystem/Pose updete k ==
  XYplot_sim : Inport
  Velocity_sim : Inport  Port=2
  Heading_sim : Inport  Port=3
  Clock : Clock
  From Workspace : FromWorkspace  VariableName=Rs_V_now  SampleTime=Ts
  From Workspace1 : FromWorkspace  VariableName=Rs_Y_now  SampleTime=Ts
  From Workspace2 : FromWorkspace  VariableName=XYplot_X  SampleTime=Ts
  From Workspace3 : FromWorkspace  VariableName=XYplot_Y  SampleTime=Ts
  Mux : Mux  Inputs=2
  Reshape : Reshape  OutputDimensionality=Customize  OutputDimensions=[pick_num,2]
  Trajectroy : Constant  Value=XYplot  VectorParams1D=off  SampleTime=-1
  Unit Delay{,1..3} (4 alike) : UnitDelay  SampleTime=Ts  HasFrameUpgradeWarning=on
  Update : MATLAB Function  TreatAsAtomicUnit=on  SystemSampleTime=Ts
      settings: RTWFcnNameOpts=Use subsystem name
  Velocity_updated : Outport  VectorParamsAs1DForOutWhenUnconnected=off
  Heading_updated : Outport  Port=2  VectorParamsAs1DForOutWhenUnconnected=off
  wires:
  XYplot_sim/1 -> Update/5(XYplot_sim), Unit Delay3/1
  Heading_sim/1 -> Unit Delay2/1, Update/9(Heading_sim)
  Clock/1 -> Update/11(Tsim)
  Velocity_sim/1 -> Update/7(Velocity_sim), Unit Delay1/1
  Update/2(Heading_updated) -> Heading_updated/1
  Update/1(Velocity_updated) -> Velocity_updated/1
  From Workspace/1 -> Update/1(Rs_V_now)
  Update/3(Heading_end) -> Unit Delay/1
  Unit Delay/1 -> Update/12(Last_Heading_end)
  From Workspace1/1 -> Update/2(Rs_Y_now)
  Unit Delay1/1 -> Update/8(Last_Velocity_sim)
  Unit Delay2/1 -> Update/10(Last_Heading_sim)
  Unit Delay3/1 -> Update/6(Last_XYplot_sim)
  Mux/1 -> Reshape/1
  From Workspace2/1 -> Mux/1
  From Workspace3/1 -> Mux/2
  Trajectroy/1 -> Update/3(XYline)
  Reshape/1 -> Update/4(XYplot)

== system ISReferenceApplication/Middle Observer3/Subsystem/VH2P ==
  Velocities : Inport
  HeadingAngles : Inport  Port=2
  Initial position : Inport  Port=3
  Iintial Velocities : Inport  Port=4
  Iintial HeadingAngles : Inport  Port=5
  Initial position1 : Inport  Port=6
  Delay1 : Delay  DelayLength=1  InitialConditionSource=Input port  InitialCondition=0  ExternalReset=Rising  SampleTime=Ts
      settings: InputPortMap=u0,r5,p4
  Delay2 : Delay  DelayLength=1  InitialConditionSource=Input port  InitialCondition=0  ExternalReset=Rising  SampleTime=Ts
      settings: InputPortMap=u0,r5,p4
  Delay3 : Delay  DelayLength=1  InitialConditionSource=Input port  InitialCondition=0  ExternalReset=Rising  SampleTime=Ts
      settings: InputPortMap=u0,r5,p4
  From Workspace : FromWorkspace  VariableName=T_sim  SampleTime=Ts
  MATLAB Function : MATLAB Function  TreatAsAtomicUnit=on
  Unit Delay3 : UnitDelay  SampleTime=Ts  HasFrameUpgradeWarning=on
  YV2P : MATLAB Function  TreatAsAtomicUnit=on  SystemSampleTime=Ts
  Position : Outport  VectorParamsAs1DForOutWhenUnconnected=off
  wires:
  MATLAB Function/1(tri) -> Delay1/2, Delay3/2, Delay2/2
  Initial position1/1 -> MATLAB Function/1(select_model)
  From Workspace/1 -> YV2P/5(Tsim), Unit Delay3/1
  Unit Delay3/1 -> YV2P/6(LastTsim)
  YV2P/1(Position) -> Position/1, Delay1/1
  Velocities/1 -> YV2P/1(Velocity), Delay3/1
  Delay3/1 -> YV2P/3(LastVelocity)
  HeadingAngles/1 -> YV2P/2(Yaw), Delay2/1
  Delay2/1 -> YV2P/4(LastYaw)
  Delay1/1 -> YV2P/7(Lastpostion)
  Initial position/1 -> Delay1/3
  Iintial Velocities/1 -> Delay3/3
  Iintial HeadingAngles/1 -> Delay2/3

== system ISReferenceApplication/Middle Observer3/Subsystem/YV_update_Np ==
  XY_sim : Inport
  Velocity_sim : Inport  Port=2
  Heading_sim : Inport  Port=3
  From Workspace1 : FromWorkspace  VariableName=T_sim  SampleTime=Ts
  From Workspace3 : FromWorkspace  VariableName=XY_Ref_Upd  SampleTime=Ts
  MATLAB Function2 : MATLAB Function  TreatAsAtomicUnit=on  SystemSampleTime=Ts
  Unit Delay1 : UnitDelay  SampleTime=Ts  HasFrameUpgradeWarning=on
  Unit Delay4 : UnitDelay  SampleTime=Ts  HasFrameUpgradeWarning=on
  Unit Delay5 : UnitDelay  SampleTime=Ts  HasFrameUpgradeWarning=on
  Velocity : Outport  VectorParamsAs1DForOutWhenUnconnected=off
  Heading angle : Outport  Port=2  VectorParamsAs1DForOutWhenUnconnected=off
  wires:
  MATLAB Function2/1(Velocity_updated) -> Velocity/1
  From Workspace3/1 -> MATLAB Function2/1(XY_ref)
  MATLAB Function2/2(Heading_updated) -> Heading angle/1
  From Workspace1/1 -> MATLAB Function2/8(Tsim)
  XY_sim/1 -> Unit Delay1/1, MATLAB Function2/2(XY_sim)
  Velocity_sim/1 -> MATLAB Function2/4(Velocity_sim), Unit Delay5/1
  Heading_sim/1 -> MATLAB Function2/6(Yaw_sim), Unit Delay4/1
  Unit Delay1/1 -> MATLAB Function2/3(LastXY_sim)
  Unit Delay5/1 -> MATLAB Function2/5(LastVelocity_sim)
  Unit Delay4/1 -> MATLAB Function2/7(LastYaw_sim)
